simulink model "opti"  (R2020a)
settings: Solver=VariableStepAuto  StartTime=0.0  StopTime=10.0  RelTol=1e-3
values from neighbouring files (symbols this model uses):
  k1 = K(1)    [ISEUfunc.m]    (also in ISEfunc.m; ITSEfunc.m; costMpfunc.m; costTr1_100Mp0func.m)
  k2 = K(2)    [ISEUfunc.m]    (also in ISEfunc.m; ITSEfunc.m; costMpfunc.m; costTr1_100Mp0func.m)
settings Model: Creator=Mertcan  LastModifiedBy=Mertcan

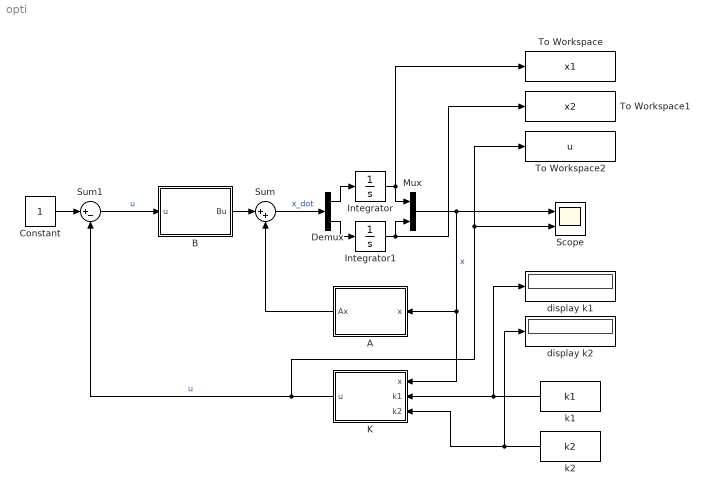
== system opti ==
  A : MATLAB Function  TreatAsAtomicUnit=on
  B : MATLAB Function  TreatAsAtomicUnit=on
  Constant : Constant
  Demux : Demux  Outputs=2
  Integrator : Integrator  InitialCondition=1
  Integrator1 : Integrator  InitialCondition=-1
  K : MATLAB Function  TreatAsAtomicUnit=on
  Mux : Mux  Inputs=2
  Scope : Scope  NumInputPorts=2
  Sum : Sum  Inputs=|++
  Sum1 : Sum  Inputs=|+-
  To Workspace : ToWorkspace  VariableName=x1  SaveFormat=Timeseries  SampleTime=-1
  To Workspace1 : ToWorkspace  VariableName=x2  SaveFormat=Timeseries  SampleTime=-1
  To Workspace2 : ToWorkspace  VariableName=u  SaveFormat=Timeseries  SampleTime=-1
  display k1 : Display
  display k2 : Display
  k1 : Constant  Value=k1
  k2 : Constant  Value=k2
  wires:
  B/1(Bu) -> Sum/1
  Mux/1 -> Scope/1, A/1(x), K/1(x)  "x"
  Sum/1 -> Demux/1  "x_dot"
  A/1(Ax) -> Sum/2
  K/1(u) -> Sum1/2, To Workspace2/1, Scope/2  "u"
  Demux/1 -> Integrator/1
  Demux/2 -> Integrator1/1
  Integrator1/1 -> To Workspace1/1, Mux/2
  Integrator/1 -> Mux/1, To Workspace/1
  k1/1 -> K/2(k1), display k1/1
  k2/1 -> K/3(k2), display k2/1
  Constant/1 -> Sum1/1
  Sum1/1 -> B/1(u)  "u"

== matlab function opti/B ==
  data: u input size=1; Bu output size=2
function Bu = B(u)

Bu = [0;u];

== matlab function opti/K ==
  data: x input size=2; u output size=1; k1 input size=1; k2 input size=1
function u = K(x,k1,k2)

u = k1*x(1) + k2*x(2);

== matlab function opti/A ==
  data: x input size=2; Ax output size=2
function Ax = A(x)

Ax = [x(2);-x(1)];
